simulink library "atr"  (Simulink 8.1)
settings: Solver=ode1  StartTime=0.0  StopTime=Inf  FixedStep=0.001  RelTol=1e-3
PostLoadFcn:
  | , if any(exist('dsrtsu_mdlpostloadfcn', 'file') == [2, 3, 6]), try dsrtsu_mdlpostloadfcn('Execute', bdroot); catch fprintf('Error in PostLoadFcn (dsrtsu_mdlpostloadfcn) for model "%s":\n %s\n', bdroot, lasterr); end, end,
undefined symbols (not defined in the file or in its folder): KACC_ACCBrakeDisableSpd_kph, KACC_BrakeRelMinSpd_kph
libraries: hcu_lib x2, csdc x1, csg x1, ctd x1, ctg x1
settings Model: DSRTSU_INTERNAL_RTI_VER=450  DSRTSU_INTERNAL_RTI_TYPE=rti1401  RTICANMMDATA=struct('GeneralSetupData',struct('modelroot','C:\Users\idiada\Desktop\HAITEC_Taiwan\trunk\AdasDragon\software\sw_development\arch\app\acc','generalsettings',struct('filesettings',struct('destfolder',struct('Name','RTICANMM_FILES','Check',1),'buildfolder',struct('Name','.','Check',1),'AbsDestfolder',struct('Name','C:\Users\idiada\Desktop\HAITEC_Taiwan\trunk\AdasDragon\software\sw_development\arch\app\acc\RTICANMM_FILES'),'AbsBuildfolder',struct('Name','C:\Users\idiada\Desktop\HAITEC_Taiwan\trunk\AdasDragon\software\sw_development\arch\app\acc'))),'options',struct('addpaths',1,'rmpaths',1,'addtrcexclusion',logical(1),'cannavigator',struct('checkmonitoring',0),'show_usrtrc',0,'use_usrtrc',0),'advanced',struct('options',[1 1 1 1 1 1 1 1 1 1 1 1 1 1 1 1 1 1 1 1 1 1 1 1 1 1 1 1 1 1 1 1 1 1 1 1 1 1 1 1 1 1 1 1 1 1 1 1 1 1 1 1 1 1 1 1 1 1 1 1 1 1 1 1 1 1 1 1 1 1 1 1 1 1 1 1 1 1 1 1 1 1 1 1 1 1 1 1 1 1 1 1 1 1 1 1 1 1 1 1]),'MPSetup',{{}},'modelname','atr','block','atr'))  DSRTSU_INTERNAL_RTIFPGA=40  Creator=AT015555  LastModifiedBy=idiada

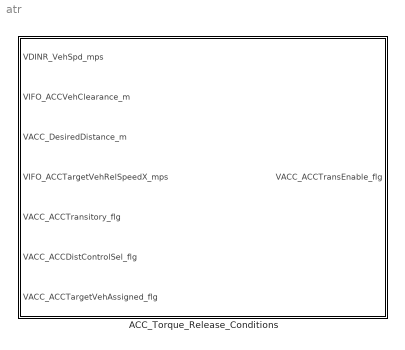
== system atr ==
  ACC_Torque_Release_Conditions : Subsystem

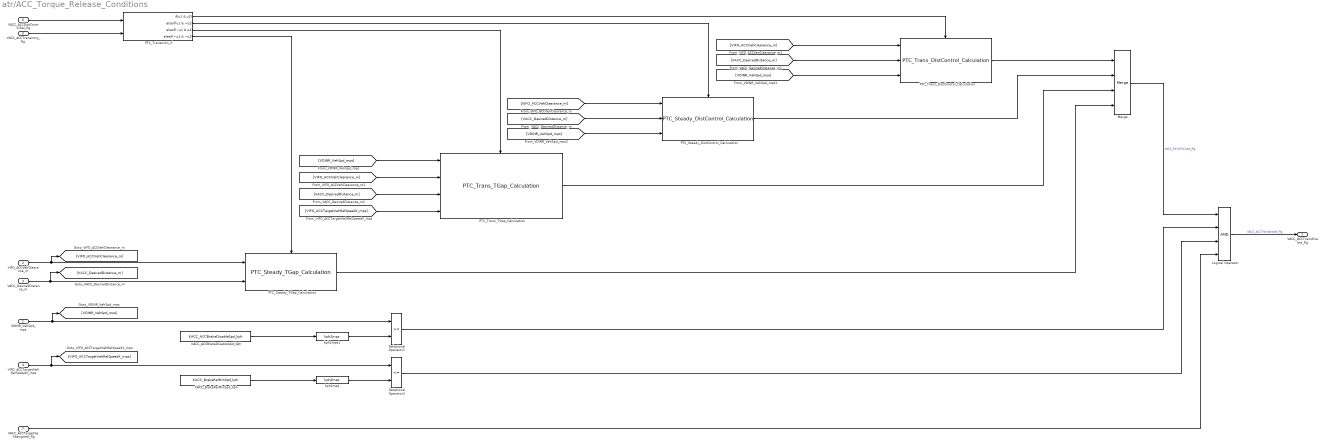
== system atr/ACC_Torque_Release_Conditions ==
  VDINR_VehSpd_mps : Inport
  VIFO_ACCVehClearance_m : Inport  Port=2
  VACC_DesiredDistance_m : Inport  Port=3
  VIFO_ACCTargetVehRelSpeedX_mps : Inport  Port=4
  VACC_ACCTransitory_flg : Inport  Port=5
  VACC_ACCDistControlSel_flg : Inport  Port=6
  VACC_ACCTargetVehAssigned_flg : Inport  Port=7
  KACC_ACCBrakeDisableSpd_kph : Constant  Value=KACC_ACCBrakeDisableSpd_kph
  KACC_BrakeRelMinSpd_kph : Constant  Value=KACC_BrakeRelMinSpd_kph
  Logical Operator : Logic  Inputs=4  AllPortsSameDT=off  OutDataTypeStr=boolean
  Merge : Merge  Inputs=4
  PTC_Steady_DistControl_Calculation : csdc/PTC_Steady_DistControl_Calculation
  PTC_Steady_TGap_Calculation : csg/PTC_Steady_TGap_Calculation
  PTC_Trans_DistControl_Calculation : ctd/PTC_Trans_DistControl_Calculation
  PTC_Trans_TGap_Calculation : ctg/PTC_Trans_TGap_Calculation
  PTC_Transition_if : If  NumInputs=2  IfExpression=u1 & u2  ElseIfExpressions=u1 & ~u2, ~u1 & u2, ~u1 & ~u2  ShowElse=off
  Relational Operator1 : RelationalOperator  OutDataTypeStr=boolean
  Relational Operator2 : RelationalOperator  Operator=<=  OutDataTypeStr=boolean
  kph2mps : hcu_lib/kph2mps
  kph2mps1 : hcu_lib/kph2mps
  VACC_ACCTransEnable_flg : Outport
  wires:
  VIFO_ACCTargetVehRelSpeedX_mps/1 -> Relational Operator2/1, [VIFO_ACCTargetVehRelSpeedX_mps]
  Logical Operator/1 -> VACC_ACCTransEnable_flg/1  "VACC_ACCTransEnable_flg"
  VACC_ACCTargetVehAssigned_flg/1 -> Logical Operator/4
  Relational Operator2/1 -> Logical Operator/3
  VDINR_VehSpd_mps/1 -> [VDINR_VehSpd_mps], Relational Operator1/1
  [VIFO_ACCTargetVehRelSpeedX_mps] -> PTC_Trans_TGap_Calculation/4
  KACC_ACCBrakeDisableSpd_kph/1 -> kph2mps1/1
  Relational Operator1/1 -> Logical Operator/2
  VACC_ACCDistControlSel_flg/1 -> PTC_Transition_if/1
  VACC_ACCTransitory_flg/1 -> PTC_Transition_if/2
  PTC_Transition_if/3 -> PTC_Trans_TGap_Calculation/Action
  [VDINR_VehSpd_mps] -> PTC_Trans_TGap_Calculation/1
  VIFO_ACCVehClearance_m/1 -> PTC_Steady_TGap_Calculation/1, [VIFO_ACCVehClearance_m]
  VACC_DesiredDistance_m/1 -> PTC_Steady_TGap_Calculation/2, [VACC_DesiredDistance_m]
  PTC_Transition_if/4 -> PTC_Steady_TGap_Calculation/Action
  PTC_Transition_if/1 -> PTC_Trans_DistControl_Calculation/Action
  PTC_Transition_if/2 -> PTC_Steady_DistControl_Calculation/Action
  [VACC_DesiredDistance_m] -> PTC_Steady_DistControl_Calculation/2
  [VIFO_ACCVehClearance_m] -> PTC_Steady_DistControl_Calculation/1
  [VIFO_ACCVehClearance_m] -> PTC_Trans_DistControl_Calculation/1
  [VACC_DesiredDistance_m] -> PTC_Trans_DistControl_Calculation/2
  [VACC_DesiredDistance_m] -> PTC_Trans_TGap_Calculation/3
  [VIFO_ACCVehClearance_m] -> PTC_Trans_TGap_Calculation/2
  PTC_Trans_DistControl_Calculation/1 -> Merge/1
  PTC_Steady_DistControl_Calculation/1 -> Merge/2
  PTC_Trans_TGap_Calculation/1 -> Merge/3
  PTC_Steady_TGap_Calculation/1 -> Merge/4
  Merge/1 -> Logical Operator/1  "VACC_PointToCoast_flg"
  [VDINR_VehSpd_mps] -> PTC_Trans_DistControl_Calculation/3
  KACC_BrakeRelMinSpd_kph/1 -> kph2mps/1
  kph2mps/1 -> Relational Operator2/2
  [VDINR_VehSpd_mps] -> PTC_Steady_DistControl_Calculation/3
  kph2mps1/1 -> Relational Operator1/2
